simulink model "MultipleAgentsChoice_NoVR"  (R2013b)
settings: Solver=ode45  StartTime=0.0  StopTime=1000  RelTol=1e-4  AbsTol=1e-4
libraries: simulink x24
(part 3 of 5)

== system MultipleAgentsChoice_NoVR/StatePropagation/SatelliteControlAccel/Agent Body3/Actual Thruster response ==
  note: UNRELIABLE THRUSTER?
  Signals : Inport
  AgentNumber : Inport  Port=2
  Bus Creator{,1..3} (4 alike) : BusCreator  Inputs=3
  Bus Creator4 : BusCreator
  Bus Selector : BusSelector  OutputSignals=A3ControlSignals,ConfigurationSignals.XValves1,ConfigurationSignals.XSwitch1,ConfigurationSignals.YValves,ConfigurationSignals.YSwitch,ConfigurationSignals.ZValves,ConfigurationSignals.ZSwitch,ConfigurationSignals.XYZValves,ConfigurationSignals.XYZSwitch,ConfigurationSignals.A3Break
  Bus Selector1 : BusSelector  OutputSignals=signal1.L1Vent,signal1.L2Vent,signal2.L1Vent,signal2.L2Vent,signal3.L1Vent,signal3.L2Vent,XYZ.L1Vent,XYZ.L2Vent  OutputAsBus=on
  Constant{,1..3} (4 alike) : Constant
  Conv2XYZ : MATLABFcn  MATLABFcn=Conv2XYZ_multi  OutputDimensions=3
  Demux : Demux
  Derivative : Derivative
  Mux : Mux  Inputs=5
  Mux1 : Mux  Inputs=2
  PressureTank : Subsystem
  Reliable : Constant
  Sum : Sum  Inputs=|++
  Switch : ManualSwitch
  ThrusterSuiteNumber1 : Constant  Value=4
  Unreliable : Constant  Value=0
  VentForce : MATLABFcn  MATLABFcn=VentForce_multi  OutputDimensions=3
  XYZthruster : Subsystem
  Xthruster : Subsystem
  Ythruster1 : Subsystem
  Zthruster1 : Subsystem
  XThrusterData : Outport
  YThrusterData : Outport  Port=2
  ZThrusterData : Outport  Port=3
  XYZThrusterData : Outport  Port=4
  Forces : Outport  Port=5
  PressureData : Outport  Port=6
  wires:
  Derivative/1 -> Mux1/2  "MainTankDerrivative"
  [NumThrusters] -> PressureTank/1(NumThrusters)
  [FeedPressure] -> XYZthruster/1(FeedPressure)
  [FeedPressure] -> Zthruster1/1(FeedPressure)
  [FeedPressure] -> Ythruster1/1(FeedPressure)
  [FeedPressure] -> Xthruster/1(FeedPressure)
  Ythruster1/3(ActivityData) -> [VentY]
  Zthruster1/3(Activitydata) -> [VentZ]
  XYZthruster/3(Activitydata) -> [VentXYZ]
  Xthruster/3(ActivityData) -> [VentX]
  [VentX] -> Bus Creator4/1
  [VentXYZ] -> Bus Creator4/4
  [VentZ] -> Bus Creator4/3
  [VentY] -> Bus Creator4/2
  ThrusterSuiteNumber1/1 -> [NumThrusters]
  PressureTank/1(TankPressure) -> Mux1/1, Derivative/1, [FeedPressure]  "MainTankPressure"
  Bus Creator4/1 -> PressureTank/2(GroupVentData), Bus Selector1/1
  Mux1/1 -> PressureData/1
  AgentNumber/1 -> Mux/5
  Constant3/1 -> Bus Creator/1
  Signals/1 -> Bus Selector/1
  Mux/1 -> Conv2XYZ/1
  Bus Selector/1 -> Demux/1  "<A3ControlSignals>"
  Demux/1 -> Xthruster/2(ForceRequest)
  Xthruster/2(Xforces) -> Mux/1
  Bus Selector/5 -> Bus Creator1/3  "<YSwitch>"
  Bus Selector/6 -> Bus Creator2/2  "<ZValves>"
  Bus Selector/7 -> Bus Creator2/3  "<ZSwitch>"
  Demux/2 -> Ythruster1/2(ForceRequest)
  Demux/3 -> Zthruster1/2(ForceRequest)
  Ythruster1/2(Yforces) -> Mux/2
  Xthruster/1(XData) -> XThrusterData/1  "A3XThrusterData"
  Ythruster1/1(YData) -> YThrusterData/1  "A3YThrusterData"
  Zthruster1/1(ZData) -> ZThrusterData/1  "A3ZThrusterData"
  Bus Creator/1 -> Xthruster/3(Data)
  Bus Selector/2 -> Bus Creator/2  "<XValves1>"
  Bus Selector/3 -> Bus Creator/3  "<XSwitch1>"
  Constant/1 -> Bus Creator1/1
  Bus Creator1/1 -> Ythruster1/3(Data)
  Constant1/1 -> Bus Creator2/1
  Bus Creator2/1 -> Zthruster1/3(Data)
  Zthruster1/2(Zforces) -> Mux/3
  Bus Selector/4 -> Bus Creator1/2  "<YValves>"
  XYZthruster/1(XYZData) -> XYZThrusterData/1  "A3XYZThrusterData"
  XYZthruster/2(XYZforces) -> Mux/4
  Demux/4 -> XYZthruster/2(ForceRequest)
  Constant2/1 -> Bus Creator3/1
  Bus Creator3/1 -> XYZthruster/3(Data)
  Bus Selector/8 -> Bus Creator3/2  "<XYZValves>"
  Bus Selector/9 -> Bus Creator3/3  "<XYZSwitch>"
  Unreliable/1 -> Switch/2
  Reliable/1 -> Switch/1
  Switch/1 -> Zthruster1/4(Reliability)
  Bus Selector/10 -> Zthruster1/5(BrokenLine)  "<A3Break>"
  VentForce/1 -> Sum/1
  Sum/1 -> Forces/1
  Conv2XYZ/1 -> Sum/2
  Bus Selector1/1 -> VentForce/1

== system MultipleAgentsChoice_NoVR/StatePropagation/SatelliteControlAccel/Agent Body3/Convert2Accels ==
  note: convert forces to accelerations based on 20kg mass and conv to km units
  Forces : Inport
  Conv KM : Gain  Gain=0.001
  mass : Gain  Gain=0.05
  Accels : Outport
  wires:
  Forces/1 -> mass/1
  Conv KM/1 -> Accels/1
  mass/1 -> Conv KM/1

== system MultipleAgentsChoice_NoVR/StatePropagation/SatelliteControlAccel/GetCmdAIL/Triggered run ==
  Trigger : TriggerPort
  DimentionsOut1 : Constant  Value=127
  GetCmdAILXYZ : MATLABFcn  MATLABFcn=GetCmdAIL  OutputDimensions=127
  Commands : Outport
  wires:
  DimentionsOut1/1 -> GetCmdAILXYZ/1
  GetCmdAILXYZ/1 -> Commands/1

== system MultipleAgentsChoice_NoVR/StatePropagation/SatelliteControlAccel/Selective Hill State Provision and Discretisation/Agent1 ==
  GEOC_Current : Inport
  LeadAgent : Inport  Port=2
  Bus Creator : BusCreator  Inputs=5
  Bus Selector2 : BusSelector  OutputSignals=Agent1Pos,Agent1Vel,Agent2Pos,Agent2Vel,Agent3Pos,Agent3Vel
  Demux : Demux  Outputs=7
  Hill State multi : MATLABFcn  MATLABFcn=HillErrors_multi  OutputDimensions=7
  Multiport Switch : MultiPortSwitch
  Mux1 : Mux  Inputs=3
  Mux2 : Mux  Inputs=3
  Mux{3..6} (4 alike) : Mux  Inputs=2
  Zero-Order Hold3 : ZeroOrderHold  SampleTime=0.5
  Zero-Order Hold4 : ZeroOrderHold  SampleTime=0.5
  Agent1 : Outport
  wires:
  Mux1/1 -> Zero-Order Hold4/1, Bus Creator/3  "HillVelCont"
  Mux2/1 -> Zero-Order Hold3/1, Bus Creator/2  "HillPosCont"
  Demux/2 -> Mux2/1
  Demux/4 -> Mux2/3
  Demux/3 -> Mux2/2
  Demux/7 -> Mux1/3
  Demux/5 -> Mux1/1
  Demux/6 -> Mux1/2
  Hill State multi/1 -> Demux/1
  LeadAgent/1 -> Multiport Switch/1
  GEOC_Current/1 -> Bus Selector2/1
  Demux/1 -> Bus Creator/1  "HillMagCont"
  Bus Creator/1 -> Agent1/1  "A1HillState"
  Mux3/1 -> Hill State multi/1
  Bus Selector2/1 -> Mux4/1  "<Agent1Pos>"
  Bus Selector2/2 -> Mux4/2  "<Agent1Vel>"
  Bus Selector2/3 -> Mux5/1  "<Agent2Pos>"
  Bus Selector2/4 -> Mux5/2  "<Agent2Vel>"
  Bus Selector2/5 -> Mux6/1  "<Agent3Pos>"
  Bus Selector2/6 -> Mux6/2  "<Agent3Vel>"
  Mux4/1 -> [Agent1]
  Mux5/1 -> [Agent2]
  Mux6/1 -> [Agent3]
  Multiport Switch/1 -> Mux3/2
  [Agent1] -> Multiport Switch/2
  [Agent2] -> Multiport Switch/3
  [Agent3] -> Multiport Switch/4
  [Agent1] -> Mux3/1
  Zero-Order Hold4/1 -> Bus Creator/5  "HillVelDisc"
  Zero-Order Hold3/1 -> Bus Creator/4  "HillPosDisc"

== system MultipleAgentsChoice_NoVR/StatePropagation/SatelliteControlAccel/Selective Hill State Provision and Discretisation/Agent2 ==
  GEOC_Current : Inport
  LeadAgent : Inport  Port=2
  Bus Creator : BusCreator  Inputs=5
  Bus Selector2 : BusSelector  OutputSignals=Agent1Pos,Agent1Vel,Agent2Pos,Agent2Vel,Agent3Pos,Agent3Vel
  Demux : Demux  Outputs=7
  Hill State multi : MATLABFcn  MATLABFcn=HillErrors_multi  OutputDimensions=7
  Multiport Switch : MultiPortSwitch
  Mux1 : Mux  Inputs=3
  Mux2 : Mux  Inputs=3
  Mux{3..6} (4 alike) : Mux  Inputs=2
  Zero-Order Hold3 : ZeroOrderHold  SampleTime=0.5
  Zero-Order Hold4 : ZeroOrderHold  SampleTime=0.5
  Agent2 : Outport
  wires:
  [Agent3] -> Multiport Switch/4
  [Agent2] -> Multiport Switch/3
  [Agent1] -> Multiport Switch/2
  Multiport Switch/1 -> Mux3/2
  Mux6/1 -> [Agent3]
  Mux5/1 -> [Agent2]
  Mux4/1 -> [Agent1]
  Bus Selector2/6 -> Mux6/2  "<Agent3Vel>"
  Bus Selector2/5 -> Mux6/1  "<Agent3Pos>"
  Bus Selector2/4 -> Mux5/2  "<Agent2Vel>"
  Bus Selector2/3 -> Mux5/1  "<Agent2Pos>"
  Bus Selector2/2 -> Mux4/2  "<Agent1Vel>"
  Bus Selector2/1 -> Mux4/1  "<Agent1Pos>"
  [Agent2] -> Mux3/1
  Mux3/1 -> Hill State multi/1
  Bus Creator/1 -> Agent2/1  "A2HillState"
  Demux/1 -> Bus Creator/1  "HillMagCont"
  GEOC_Current/1 -> Bus Selector2/1
  LeadAgent/1 -> Multiport Switch/1
  Hill State multi/1 -> Demux/1
  Demux/6 -> Mux1/2
  Demux/5 -> Mux1/1
  Demux/7 -> Mux1/3
  Demux/3 -> Mux2/2
  Demux/4 -> Mux2/3
  Demux/2 -> Mux2/1
  Mux2/1 -> Zero-Order Hold3/1, Bus Creator/2  "HillPosCont"
  Mux1/1 -> Zero-Order Hold4/1, Bus Creator/3  "HillVelCont"
  Zero-Order Hold3/1 -> Bus Creator/4  "HillPosDisc"
  Zero-Order Hold4/1 -> Bus Creator/5  "HillVelDisc"

== system MultipleAgentsChoice_NoVR/StatePropagation/SatelliteControlAccel/Selective Hill State Provision and Discretisation/Agent3 ==
  GEOC_Current : Inport
  LeadAgent : Inport  Port=2
  Bus Creator : BusCreator  Inputs=5
  Bus Selector2 : BusSelector  OutputSignals=Agent1Pos,Agent1Vel,Agent2Pos,Agent2Vel,Agent3Pos,Agent3Vel
  Demux : Demux  Outputs=7
  Hill State multi : MATLABFcn  MATLABFcn=HillErrors_multi  OutputDimensions=7
  Multiport Switch : MultiPortSwitch
  Mux1 : Mux  Inputs=3
  Mux2 : Mux  Inputs=3
  Mux{3..6} (4 alike) : Mux  Inputs=2
  Zero-Order Hold3 : ZeroOrderHold  SampleTime=0.5
  Zero-Order Hold4 : ZeroOrderHold  SampleTime=0.5
  Agent3 : Outport
  wires:
  Mux1/1 -> Zero-Order Hold4/1, Bus Creator/3  "HillVelCont"
  Mux2/1 -> Zero-Order Hold3/1, Bus Creator/2  "HillPosCont"
  Demux/2 -> Mux2/1
  Demux/4 -> Mux2/3
  Demux/3 -> Mux2/2
  Demux/7 -> Mux1/3
  Demux/5 -> Mux1/1
  Demux/6 -> Mux1/2
  Hill State multi/1 -> Demux/1
  LeadAgent/1 -> Multiport Switch/1
  GEOC_Current/1 -> Bus Selector2/1
  Zero-Order Hold4/1 -> Bus Creator/5  "HillVelDisc"
  Demux/1 -> Bus Creator/1  "HillMagCont"
  Bus Creator/1 -> Agent3/1  "A3HillState"
  Mux3/1 -> Hill State multi/1
  Bus Selector2/1 -> Mux4/1  "<Agent1Pos>"
  Bus Selector2/2 -> Mux4/2  "<Agent1Vel>"
  Bus Selector2/3 -> Mux5/1  "<Agent2Pos>"
  Bus Selector2/4 -> Mux5/2  "<Agent2Vel>"
  Bus Selector2/5 -> Mux6/1  "<Agent3Pos>"
  Bus Selector2/6 -> Mux6/2  "<Agent3Vel>"
  Mux4/1 -> [Agent1]
  Mux5/1 -> [Agent2]
  Mux6/1 -> [Agent3]
  [Agent1] -> Multiport Switch/2
  [Agent2] -> Multiport Switch/3
  [Agent3] -> Multiport Switch/4
  [Agent3] -> Mux3/1
  Multiport Switch/1 -> Mux3/2
  Zero-Order Hold3/1 -> Bus Creator/4  "HillPosDisc"

== system MultipleAgentsChoice_NoVR/StatePropagation/SatelliteControlAccel/Selective Hill State Provision and Discretisation/MemoryUpdate ==
  GEOC_Current : Inport
  LeadAgent : Inport  Port=2
  Bus Selector2 : BusSelector  OutputSignals=Agent1Pos,Agent1Vel,Agent2Pos,Agent2Vel,Agent3Pos,Agent3Vel
  Multiport Switch : MultiPortSwitch
  Mux4 : Mux  Inputs=2
  Mux5 : Mux  Inputs=2
  Mux6 : Mux  Inputs=2
  Updatememory : MATLABFcn  MATLABFcn=UpdateMemory  OutputDimensions=0
  wires:
  Multiport Switch/1 -> Updatememory/1
  Mux6/1 -> Multiport Switch/4
  Mux5/1 -> Multiport Switch/3
  Mux4/1 -> Multiport Switch/2
  Bus Selector2/6 -> Mux6/2  "<Agent3Vel>"
  Bus Selector2/5 -> Mux6/1  "<Agent3Pos>"
  Bus Selector2/4 -> Mux5/2  "<Agent2Vel>"
  Bus Selector2/3 -> Mux5/1  "<Agent2Pos>"
  Bus Selector2/2 -> Mux4/2  "<Agent1Vel>"
  Bus Selector2/1 -> Mux4/1  "<Agent1Pos>"
  GEOC_Current/1 -> Bus Selector2/1
  LeadAgent/1 -> Multiport Switch/1

== system MultipleAgentsChoice_NoVR/StatePropagation/SatelliteControlAccel/TriggeredSendAgent/SendToAIL ==
  A1ActualForces : Inport
  A1PlanMsg : Inport  Port=2
  A1DesiredForces : Inport  Port=3
  A1StateInfo : Inport  Port=4
  A1tank : Inport  Port=5
  A1XThruster : Inport  Port=6
  A1YThruster : Inport  Port=7
  A1ZThruster : Inport  Port=8
  A1XYZThruster : Inport  Port=9
  A2ActualForces : Inport  Port=10
  A2PlanMsg : Inport  Port=11
  A2DesiredForces : Inport  Port=12
  A2StateInfo : Inport  Port=13
  A2tank : Inport  Port=14
  A2XThruster : Inport  Port=15
  A2YThruster : Inport  Port=16
  A2ZThruster : Inport  Port=17
  A2XYZThruster : Inport  Port=18
  A3ActualForces : Inport  Port=19
  A3PlanMsg : Inport  Port=20
  A3DesiredForces : Inport  Port=21
  A3StateInfo : Inport  Port=22
  A3tank : Inport  Port=23
  A3XThruster : Inport  Port=24
  A3YThruster : Inport  Port=25
  A3ZThruster : Inport  Port=26
  A3XYZThruster : Inport  Port=27
  Display : Display
  MATLAB Fcn : MATLABFcn  MATLABFcn=CommunicateWithTagsMulti  OutputDimensions=0
  Mux : Mux  Inputs=27
  wires:
  A1ActualForces/1 -> Mux/1  "A1ActualForces"
  A1PlanMsg/1 -> Mux/2  "A1PlanMsg"
  A1StateInfo/1 -> Mux/4  "A1StateInfo"
  A1XThruster/1 -> Mux/6  "A1XThruster"
  A1YThruster/1 -> Mux/7  "A1YThruster"
  A1ZThruster/1 -> Mux/8  "A1ZThruster"
  A1DesiredForces/1 -> Mux/3  "A1DesiredForfces"
  A1tank/1 -> Mux/5  "A1Tank"
  A2ActualForces/1 -> Mux/10  "A2ActualForces"
  A2PlanMsg/1 -> Mux/11  "A2PlanMsg"
  A2StateInfo/1 -> Mux/13  "A2StateInfo"
  A2XThruster/1 -> Mux/15  "A2XThruster"
  A2YThruster/1 -> Mux/16  "A2YThruster"
  A2ZThruster/1 -> Mux/17  "A2ZThruster"
  A2DesiredForces/1 -> Mux/12  "A2DesiredForces"
  A2tank/1 -> Mux/14  "A2Tank"
  A1XYZThruster/1 -> Mux/9  "A1XYZThruster"
  A2XYZThruster/1 -> Mux/18  "A2XYZThruster"
  A3PlanMsg/1 -> Mux/20  "A3PlanMsg"
  A3DesiredForces/1 -> Mux/21  "A3DesiredForces"
  A3StateInfo/1 -> Mux/22  "A3StateInfo"
  A3tank/1 -> Mux/23  "A3Tank"
  A3XThruster/1 -> Mux/24  "A3XThruster"
  A3YThruster/1 -> Mux/25  "A3YThruster"
  A3ZThruster/1 -> Mux/26  "A3ZThruster"
  A3XYZThruster/1 -> Mux/27  "A3XYZThruster"
  A3ActualForces/1 -> Mux/19  "A3ActualForces"
  Mux/1 -> MATLAB Fcn/1, Display/1

== system MultipleAgentsChoice_NoVR/StatePropagation/SatelliteControlAccel/TriggeredSendCont/SendToCont ==
  A1ActualForces : Inport
  A1PlanMsg : Inport  Port=2
  A1DesiredForces : Inport  Port=3
  A1StateInfo : Inport  Port=4
  A1tank : Inport  Port=5
  A1XThruster : Inport  Port=6
  A1YThruster : Inport  Port=7
  A1ZThruster : Inport  Port=8
  A1XYZThruster : Inport  Port=9
  A2ActualForces : Inport  Port=10
  A2PlanMsg : Inport  Port=11
  A2DesiredForces : Inport  Port=12
  A2StateInfo : Inport  Port=13
  A2tank : Inport  Port=14
  A2XThruster : Inport  Port=15
  A2YThruster : Inport  Port=16
  A2ZThruster : Inport  Port=17
  A2XYZThruster : Inport  Port=18
  A3ActualForces : Inport  Port=19
  A3PlanMsg : Inport  Port=20
  A3DesiredForces : Inport  Port=21
  A3StateInfo : Inport  Port=22
  A3tank : Inport  Port=23
  A3XThruster : Inport  Port=24
  A3YThruster : Inport  Port=25
  A3ZThruster : Inport  Port=26
  A3XYZThruster : Inport  Port=27
  Display : Display
  MATLAB Fcn : MATLABFcn  MATLABFcn=CommunicateWithCont  OutputDimensions=0
  Mux : Mux  Inputs=27
  wires:
  Mux/1 -> Display/1, MATLAB Fcn/1
  A3ActualForces/1 -> Mux/19  "A3ActualForces"
  A3XYZThruster/1 -> Mux/27  "A3XYZThruster"
  A3ZThruster/1 -> Mux/26  "A3ZThruster"
  A3YThruster/1 -> Mux/25  "A3YThruster"
  A3XThruster/1 -> Mux/24  "A3XThruster"
  A3tank/1 -> Mux/23  "A3tank"
  A3StateInfo/1 -> Mux/22  "A3StateInfo"
  A3DesiredForces/1 -> Mux/21  "A3DesiredForces"
  A3PlanMsg/1 -> Mux/20  "A3PlanMsg"
  A2XYZThruster/1 -> Mux/18  "A2XYZThruster"
  A1XYZThruster/1 -> Mux/9  "A1XYZThruster"
  A2tank/1 -> Mux/14  "A2tank"
  A2DesiredForces/1 -> Mux/12  "A2DesiredForces"
  A2ZThruster/1 -> Mux/17  "A2ZThruster"
  A2YThruster/1 -> Mux/16  "A2YThruster"
  A2XThruster/1 -> Mux/15  "A2XThruster"
  A2StateInfo/1 -> Mux/13  "A2StateInfo"
  A2PlanMsg/1 -> Mux/11  "A2PlanMsg"
  A2ActualForces/1 -> Mux/10  "A2ActualForces"
  A1tank/1 -> Mux/5  "A1tank"
  A1DesiredForces/1 -> Mux/3  "A1DesiredForfces"
  A1ZThruster/1 -> Mux/8  "A1ZThruster"
  A1YThruster/1 -> Mux/7  "A1YThruster"
  A1XThruster/1 -> Mux/6  "A1XThruster"
  A1StateInfo/1 -> Mux/4  "A1StateInfo"
  A1PlanMsg/1 -> Mux/2  "A1PlanMsg"
  A1ActualForces/1 -> Mux/1  "A1ActualForces"

== system MultipleAgentsChoice_NoVR/StatePropagation/SatelliteControlAccel/Agent Body1/Actual Thruster response/PressureTank ==
  NumThrusters : Inport
  GroupVentData : Inport  Port=2
  Clock : Clock
  Display : Display
  DropRate : MATLABFcn  MATLABFcn=DropRate_multi  OutputDimensions=1
  Integrator : Integrator  InitialConditionSource=external
  Mux : Mux  Inputs=2
  Start : Constant  Value=0
  StartPressure : Constant  Value=100
  Switch1 : Switch
  TankPressure : Outport
  wires:
  DropRate/1 -> Switch1/1
  Mux/1 -> DropRate/1
  NumThrusters/1 -> Mux/1
  GroupVentData/1 -> Mux/2
  Switch1/1 -> Integrator/1
  Clock/1 -> Switch1/2
  Start/1 -> Switch1/3
  Integrator/1 -> Display/1, TankPressure/1
  StartPressure/1 -> Integrator/2

== system MultipleAgentsChoice_NoVR/StatePropagation/SatelliteControlAccel/Agent Body1/Actual Thruster response/XYZthruster ==
  note: NB:-Agent has no knowledge of red blocks
      |             -Blue blocks prescribed by agent
  note: Tank pressure and thruster selection: must declare number of thrusters
  FeedPressure : Inport
  ForceRequest : Inport  Port=2
  Data : Inport  Port=3
  Bus Creator2 : BusCreator  Inputs=3
  Bus Selector : BusSelector  OutputSignals=XYZValves,XYZSwitch
  Constant : Constant
  Constant1 : Constant  Value=0
  Switch : Switch  Criteria=u2 ~= 0
  Thruster1 : Subsystem
  XYZData : Outport
  XYZforces : Outport  Port=2
  Activitydata : Outport  Port=3
  wires:
  ForceRequest/1 -> Thruster1/4(ForceRequest)  "XYZforces"
  Thruster1/1(L1Vent) -> Bus Creator2/1  "L1Vent"
  Thruster1/2(L2Vent) -> Bus Creator2/2  "L2Vent"
  FeedPressure/1 -> Thruster1/2(FeedPressure)
  Constant/1 -> Switch/1
  Constant1/1 -> Switch/3
  Thruster1/4(thrusterData) -> XYZData/1  "A1TXYZ1"
  Data/1 -> Bus Selector/1
  Bus Selector/1 -> Thruster1/1(ValveAssign)  "<XYZValves>"
  Bus Selector/2 -> Thruster1/3(MainSwitch)  "<XYZSwitch>"
  Thruster1/3(Forces) -> XYZforces/1, Switch/2
  Switch/1 -> Bus Creator2/3  "Active1"
  Bus Creator2/1 -> Activitydata/1  "XYZ"

== system MultipleAgentsChoice_NoVR/StatePropagation/SatelliteControlAccel/Agent Body1/Actual Thruster response/Xthruster ==
  note: Tank pressure and thruster selection: must declare number of thrusters
  note: NB:-Agent has no knowledge of red blocks
      |             -Blue blocks prescribed by agent
  FeedPressure : Inport
  ForceRequest : Inport  Port=2
  Data : Inport  Port=3
  Bus Creator2 : BusCreator  Inputs=3
  Bus Selector : BusSelector  OutputSignals=XValves1,XSwitch1
  Constant : Constant
  Constant1 : Constant  Value=0
  Switch : Switch  Criteria=u2 ~= 0
  Thruster1 : Subsystem
  XData : Outport
  Xforces : Outport  Port=2
  ActivityData : Outport  Port=3
  wires:
  Bus Creator2/1 -> ActivityData/1
  Switch/1 -> Bus Creator2/3  "Active1"
  Thruster1/3(Forces) -> Xforces/1, Switch/2
  Bus Selector/2 -> Thruster1/3(MainSwitch)  "<XSwitch1>"
  Bus Selector/1 -> Thruster1/1(ValveAssign)  "<XValves1>"
  Data/1 -> Bus Selector/1
  Thruster1/4(ThrusterData) -> XData/1
  Constant1/1 -> Switch/3
  Constant/1 -> Switch/1
  FeedPressure/1 -> Thruster1/2(FeedPressure)
  Thruster1/2(L2Vent) -> Bus Creator2/2  "L2Vent"
  Thruster1/1(L1Vent) -> Bus Creator2/1  "L1Vent"
  ForceRequest/1 -> Thruster1/4(ForceRequest)  "Xforces"

== system MultipleAgentsChoice_NoVR/StatePropagation/SatelliteControlAccel/Agent Body1/Actual Thruster response/Ythruster1 ==
  note: NB:-Agent has no knowledge of red blocks
      |             -Blue blocks prescribed by agent
  note: Tank pressure and thruster selection: must declare number of thrusters
  FeedPressure : Inport
  ForceRequest : Inport  Port=2
  Data : Inport  Port=3
  Bus Creator2 : BusCreator  Inputs=3
  Bus Selector : BusSelector  OutputSignals=YValves,YSwitch
  Constant : Constant
  Constant1 : Constant  Value=0
  Switch : Switch  Criteria=u2 ~= 0
  Thruster1 : Subsystem
  YData : Outport
  Yforces : Outport  Port=2
  ActivityData : Outport  Port=3
  wires:
  ForceRequest/1 -> Thruster1/4(ForceRequest)  "Yforces"
  Thruster1/1(L1Vent) -> Bus Creator2/1  "L1Vent"
  Thruster1/2(L2Vent) -> Bus Creator2/2  "L2Vent"
  [ValveAssign1] -> Thruster1/1(ValveAssign)
  [MainSwitch1] -> Thruster1/3(MainSwitch)
  FeedPressure/1 -> Thruster1/2(FeedPressure)
  Constant/1 -> Switch/1
  Constant1/1 -> Switch/3
  Thruster1/4(thrusterData) -> YData/1  "A1TY1"
  Data/1 -> Bus Selector/1
  Bus Selector/1 -> [ValveAssign1]  "<YValves>"
  Bus Selector/2 -> [MainSwitch1]  "<YSwitch>"
  Thruster1/3(Forces) -> Yforces/1, Switch/2
  Switch/1 -> Bus Creator2/3  "Active1"
  Bus Creator2/1 -> ActivityData/1

== system MultipleAgentsChoice_NoVR/StatePropagation/SatelliteControlAccel/Agent Body1/Actual Thruster response/Zthruster1 ==
  note: Tank pressure and thruster selection: must declare number of thrusters
  note: NB:-Agent has no knowledge of red blocks
      |             -Blue blocks prescribed by agent
  FeedPressure : Inport
  ForceRequest : Inport  Port=2
  Data : Inport  Port=3
  Reliability : Inport  Port=4
  BrokenLine : Inport  Port=5
  Bus Creator2 : BusCreator  Inputs=3
  Bus Selector : BusSelector  OutputSignals=ZValves,ZSwitch
  Constant : Constant
  Constant1 : Constant  Value=0
  Switch : Switch  Criteria=u2 ~= 0
  Thruster1 : Subsystem
  ZData : Outport
  Zforces : Outport  Port=2
  Activitydata : Outport  Port=3
  wires:
  Reliability/1 -> Thruster1/5(Reliability)
  Bus Creator2/1 -> Activitydata/1
  Switch/1 -> Bus Creator2/3  "Active1"
  Thruster1/3(Forces) -> Switch/2, Zforces/1
  Bus Selector/2 -> Thruster1/3(MainSwitch)  "<ZSwitch>"
  Bus Selector/1 -> Thruster1/1(ValveAssign)  "<ZValves>"
  Data/1 -> Bus Selector/1
  Thruster1/4(thrusterData) -> ZData/1  "A1TZ1"
  Constant1/1 -> Switch/3
  Constant/1 -> Switch/1
  FeedPressure/1 -> Thruster1/2(FeedPressure)
  Thruster1/2(L2Vent) -> Bus Creator2/2  "L2Vent"
  Thruster1/1(L1Vent) -> Bus Creator2/1  "L1Vent"
  ForceRequest/1 -> Thruster1/4(ForceRequest)  "Zforces"
  BrokenLine/1 -> Thruster1/6(BrokenLine)

== system MultipleAgentsChoice_NoVR/StatePropagation/SatelliteControlAccel/Agent Body2/Actual Thruster response/PressureTank ==
  NumThrusters : Inport
  GroupVentData : Inport  Port=2
  Clock : Clock
  Display : Display
  DropRate : MATLABFcn  MATLABFcn=DropRate_multi  OutputDimensions=1
  Integrator : Integrator  InitialConditionSource=external
  Mux : Mux  Inputs=2
  Start : Constant  Value=0
  StartPressure : Constant  Value=100
  Switch1 : Switch
  TankPressure : Outport
  wires:
  StartPressure/1 -> Integrator/2
  Integrator/1 -> TankPressure/1, Display/1
  Start/1 -> Switch1/3
  Clock/1 -> Switch1/2
  Switch1/1 -> Integrator/1
  GroupVentData/1 -> Mux/2
  NumThrusters/1 -> Mux/1
  Mux/1 -> DropRate/1
  DropRate/1 -> Switch1/1

== system MultipleAgentsChoice_NoVR/StatePropagation/SatelliteControlAccel/Agent Body2/Actual Thruster response/XYZthruster ==
  note: Tank pressure and thruster selection: must declare number of thrusters
  note: NB:-Agent has no knowledge of red blocks
      |             -Blue blocks prescribed by agent
  FeedPressure : Inport
  ForceRequest : Inport  Port=2
  Data : Inport  Port=3
  Bus Creator2 : BusCreator  Inputs=3
  Bus Selector : BusSelector  OutputSignals=XYZValves,XYZSwitch
  Constant : Constant
  Constant1 : Constant  Value=0
  Switch : Switch  Criteria=u2 ~= 0
  Thruster1 : Subsystem
  XYZData : Outport
  XYZforces : Outport  Port=2
  Activitydata : Outport  Port=3
  wires:
  Bus Creator2/1 -> Activitydata/1  "XYZ"
  Switch/1 -> Bus Creator2/3  "Active1"
  Thruster1/3(Forces) -> Switch/2, XYZforces/1
  Bus Selector/2 -> Thruster1/3(MainSwitch)  "<XYZSwitch>"
  Bus Selector/1 -> Thruster1/1(ValveAssign)  "<XYZValves>"
  Data/1 -> Bus Selector/1
  Thruster1/4(thrusterData) -> XYZData/1
  Constant1/1 -> Switch/3
  Constant/1 -> Switch/1
  FeedPressure/1 -> Thruster1/2(FeedPressure)
  Thruster1/2(L2Vent) -> Bus Creator2/2  "L2Vent"
  Thruster1/1(L1Vent) -> Bus Creator2/1  "L1Vent"
  ForceRequest/1 -> Thruster1/4(ForceRequest)  "XYZforces"

== system MultipleAgentsChoice_NoVR/StatePropagation/SatelliteControlAccel/Agent Body2/Actual Thruster response/Xthruster ==
  note: NB:-Agent has no knowledge of red blocks
      |             -Blue blocks prescribed by agent
  note: Tank pressure and thruster selection: must declare number of thrusters
  FeedPressure : Inport
  ForceRequest : Inport  Port=2
  Data : Inport  Port=3
  Bus Creator2 : BusCreator  Inputs=3
  Bus Selector : BusSelector  OutputSignals=XValves1,XSwitch1
  Constant : Constant
  Constant1 : Constant  Value=0
  Switch : Switch  Criteria=u2 ~= 0
  Thruster1 : Subsystem
  XData : Outport
  Xforces : Outport  Port=2
  ActivityData : Outport  Port=3
  wires:
  ForceRequest/1 -> Thruster1/4(ForceRequest)  "Xforces"
  Thruster1/1(L1Vent) -> Bus Creator2/1  "L1Vent"
  Thruster1/2(L2Vent) -> Bus Creator2/2  "L2Vent"
  FeedPressure/1 -> Thruster1/2(FeedPressure)
  Constant/1 -> Switch/1
  Constant1/1 -> Switch/3
  Thruster1/4(ThrusterData) -> XData/1  "A2TX"
  Data/1 -> Bus Selector/1
  Bus Selector/1 -> Thruster1/1(ValveAssign)  "<XValves1>"
  Bus Selector/2 -> Thruster1/3(MainSwitch)  "<XSwitch1>"
  Thruster1/3(Forces) -> Switch/2, Xforces/1
  Switch/1 -> Bus Creator2/3  "Active1"
  Bus Creator2/1 -> ActivityData/1

== system MultipleAgentsChoice_NoVR/StatePropagation/SatelliteControlAccel/Agent Body2/Actual Thruster response/Ythruster1 ==
  note: Tank pressure and thruster selection: must declare number of thrusters
  note: NB:-Agent has no knowledge of red blocks
      |             -Blue blocks prescribed by agent
  FeedPressure : Inport
  ForceRequest : Inport  Port=2
  Data : Inport  Port=3
  Bus Creator2 : BusCreator  Inputs=3
  Bus Selector : BusSelector  OutputSignals=YValves,YSwitch
  Constant : Constant
  Constant1 : Constant  Value=0
  Switch : Switch  Criteria=u2 ~= 0
  Thruster1 : Subsystem
  YData : Outport
  Yforces : Outport  Port=2
  ActivityData : Outport  Port=3
  wires:
  Bus Creator2/1 -> ActivityData/1
  Switch/1 -> Bus Creator2/3  "Active1"
  Thruster1/3(Forces) -> Switch/2, Yforces/1
  Bus Selector/2 -> [MainSwitch1]  "<YSwitch>"
  Bus Selector/1 -> [ValveAssign1]  "<YValves>"
  Data/1 -> Bus Selector/1
  Thruster1/4(thrusterData) -> YData/1  "A2TY"
  Constant1/1 -> Switch/3
  Constant/1 -> Switch/1
  FeedPressure/1 -> Thruster1/2(FeedPressure)
  [MainSwitch1] -> Thruster1/3(MainSwitch)
  [ValveAssign1] -> Thruster1/1(ValveAssign)
  Thruster1/2(L2Vent) -> Bus Creator2/2  "L2Vent"
  Thruster1/1(L1Vent) -> Bus Creator2/1  "L1Vent"
  ForceRequest/1 -> Thruster1/4(ForceRequest)  "Yforces"

== system MultipleAgentsChoice_NoVR/StatePropagation/SatelliteControlAccel/Agent Body2/Actual Thruster response/Zthruster1 ==
  note: NB:-Agent has no knowledge of red blocks
      |             -Blue blocks prescribed by agent
  note: Tank pressure and thruster selection: must declare number of thrusters
  FeedPressure : Inport
  ForceRequest : Inport  Port=2
  Data : Inport  Port=3
  Reliability : Inport  Port=4
  BrokenLine : Inport  Port=5
  Bus Creator2 : BusCreator  Inputs=3
  Bus Selector : BusSelector  OutputSignals=ZValves,ZSwitch
  Constant : Constant
  Constant1 : Constant  Value=0
  Switch : Switch  Criteria=u2 ~= 0
  Thruster1 : Subsystem
  ZData : Outport
  Zforces : Outport  Port=2
  Activitydata : Outport  Port=3
  wires:
  ForceRequest/1 -> Thruster1/4(ForceRequest)  "Zforces"
  Thruster1/1(L1Vent) -> Bus Creator2/1  "L1Vent"
  Thruster1/2(L2Vent) -> Bus Creator2/2  "L2Vent"
  FeedPressure/1 -> Thruster1/2(FeedPressure)
  Constant/1 -> Switch/1
  Constant1/1 -> Switch/3
  Thruster1/4(thrusterData) -> ZData/1  "A2TZ"
  Data/1 -> Bus Selector/1
  Bus Selector/1 -> Thruster1/1(ValveAssign)  "<ZValves>"
  Bus Selector/2 -> Thruster1/3(MainSwitch)  "<ZSwitch>"
  Thruster1/3(Forces) -> Zforces/1, Switch/2
  Switch/1 -> Bus Creator2/3  "Active1"
  Bus Creator2/1 -> Activitydata/1
  Reliability/1 -> Thruster1/5(Reliability)
  BrokenLine/1 -> Thruster1/6(BrokenLine)

== system MultipleAgentsChoice_NoVR/StatePropagation/SatelliteControlAccel/Agent Body3/Actual Thruster response/PressureTank ==
  NumThrusters : Inport
  GroupVentData : Inport  Port=2
  Clock : Clock
  Display : Display
  DropRate : MATLABFcn  MATLABFcn=DropRate_multi  OutputDimensions=1
  Integrator : Integrator  InitialConditionSource=external
  Mux : Mux  Inputs=2
  Start : Constant  Value=0
  StartPressure : Constant  Value=100
  Switch1 : Switch
  TankPressure : Outport
  wires:
  StartPressure/1 -> Integrator/2
  Integrator/1 -> TankPressure/1, Display/1
  Start/1 -> Switch1/3
  Clock/1 -> Switch1/2
  Switch1/1 -> Integrator/1
  GroupVentData/1 -> Mux/2
  NumThrusters/1 -> Mux/1
  Mux/1 -> DropRate/1
  DropRate/1 -> Switch1/1

== system MultipleAgentsChoice_NoVR/StatePropagation/SatelliteControlAccel/Agent Body3/Actual Thruster response/XYZthruster ==
  note: Tank pressure and thruster selection: must declare number of thrusters
  note: NB:-Agent has no knowledge of red blocks
      |             -Blue blocks prescribed by agent
  FeedPressure : Inport
  ForceRequest : Inport  Port=2
  Data : Inport  Port=3
  Bus Creator2 : BusCreator  Inputs=3
  Bus Selector : BusSelector  OutputSignals=XYZValves,XYZSwitch
  Constant : Constant
  Constant1 : Constant  Value=0
  Switch : Switch  Criteria=u2 ~= 0
  Thruster1 : Subsystem
  XYZData : Outport
  XYZforces : Outport  Port=2
  Activitydata : Outport  Port=3
  wires:
  Bus Creator2/1 -> Activitydata/1  "XYZ"
  Switch/1 -> Bus Creator2/3  "Active1"
  Thruster1/3(Forces) -> Switch/2, XYZforces/1
  Bus Selector/2 -> Thruster1/3(MainSwitch)  "<XYZSwitch>"
  Bus Selector/1 -> Thruster1/1(ValveAssign)  "<XYZValves>"
  Data/1 -> Bus Selector/1
  Thruster1/4(thrusterData) -> XYZData/1  "A3TXYZ"
  Constant1/1 -> Switch/3
  Constant/1 -> Switch/1
  FeedPressure/1 -> Thruster1/2(FeedPressure)
  Thruster1/2(L2Vent) -> Bus Creator2/2  "L2Vent"
  Thruster1/1(L1Vent) -> Bus Creator2/1  "L1Vent"
  ForceRequest/1 -> Thruster1/4(ForceRequest)  "XYZforces"

== system MultipleAgentsChoice_NoVR/StatePropagation/SatelliteControlAccel/Agent Body3/Actual Thruster response/Xthruster ==
  note: NB:-Agent has no knowledge of red blocks
      |             -Blue blocks prescribed by agent
  note: Tank pressure and thruster selection: must declare number of thrusters
  FeedPressure : Inport
  ForceRequest : Inport  Port=2
  Data : Inport  Port=3
  Bus Creator2 : BusCreator  Inputs=3
  Bus Selector : BusSelector  OutputSignals=XValves1,XSwitch1
  Constant : Constant
  Constant1 : Constant  Value=0
  Switch : Switch  Criteria=u2 ~= 0
  Thruster1 : Subsystem
  XData : Outport
  Xforces : Outport  Port=2
  ActivityData : Outport  Port=3
  wires:
  ForceRequest/1 -> Thruster1/4(ForceRequest)  "Xforces"
  Thruster1/1(L1Vent) -> Bus Creator2/1  "L1Vent"
  Thruster1/2(L2Vent) -> Bus Creator2/2  "L2Vent"
  FeedPressure/1 -> Thruster1/2(FeedPressure)
  Constant/1 -> Switch/1
  Constant1/1 -> Switch/3
  Thruster1/4(ThrusterData) -> XData/1  "A3TX"
  Data/1 -> Bus Selector/1
  Bus Selector/1 -> Thruster1/1(ValveAssign)  "<XValves1>"
  Bus Selector/2 -> Thruster1/3(MainSwitch)  "<XSwitch1>"
  Thruster1/3(Forces) -> Switch/2, Xforces/1
  Switch/1 -> Bus Creator2/3  "Active1"
  Bus Creator2/1 -> ActivityData/1

== system MultipleAgentsChoice_NoVR/StatePropagation/SatelliteControlAccel/Agent Body3/Actual Thruster response/Ythruster1 ==
  note: Tank pressure and thruster selection: must declare number of thrusters
  note: NB:-Agent has no knowledge of red blocks
      |             -Blue blocks prescribed by agent
  FeedPressure : Inport
  ForceRequest : Inport  Port=2
  Data : Inport  Port=3
  Bus Creator2 : BusCreator  Inputs=3
  Bus Selector : BusSelector  OutputSignals=YValves,YSwitch
  Constant : Constant
  Constant1 : Constant  Value=0
  Switch : Switch  Criteria=u2 ~= 0
  Thruster1 : Subsystem
  YData : Outport
  Yforces : Outport  Port=2
  ActivityData : Outport  Port=3
  wires:
  Bus Creator2/1 -> ActivityData/1
  Switch/1 -> Bus Creator2/3  "Active1"
  Thruster1/3(Forces) -> Switch/2, Yforces/1
  Bus Selector/2 -> [MainSwitch1]  "<YSwitch>"
  Bus Selector/1 -> [ValveAssign1]  "<YValves>"
  Data/1 -> Bus Selector/1
  Thruster1/4(thrusterData) -> YData/1  "A3TY"
  Constant1/1 -> Switch/3
  Constant/1 -> Switch/1
  FeedPressure/1 -> Thruster1/2(FeedPressure)
  [MainSwitch1] -> Thruster1/3(MainSwitch)
  [ValveAssign1] -> Thruster1/1(ValveAssign)
  Thruster1/2(L2Vent) -> Bus Creator2/2  "L2Vent"
  Thruster1/1(L1Vent) -> Bus Creator2/1  "L1Vent"
  ForceRequest/1 -> Thruster1/4(ForceRequest)  "Yforces"

== system MultipleAgentsChoice_NoVR/StatePropagation/SatelliteControlAccel/Agent Body3/Actual Thruster response/Zthruster1 ==
  note: NB:-Agent has no knowledge of red blocks
      |             -Blue blocks prescribed by agent
  note: Tank pressure and thruster selection: must declare number of thrusters
  FeedPressure : Inport
  ForceRequest : Inport  Port=2
  Data : Inport  Port=3
  Reliability : Inport  Port=4
  BrokenLine : Inport  Port=5
  Bus Creator2 : BusCreator  Inputs=3
  Bus Selector : BusSelector  OutputSignals=ZValves,ZSwitch
  Constant : Constant
  Constant1 : Constant  Value=0
  Switch : Switch  Criteria=u2 ~= 0
  Thruster1 : Subsystem
  ZData : Outport
  Zforces : Outport  Port=2
  Activitydata : Outport  Port=3
  wires:
  ForceRequest/1 -> Thruster1/4(ForceRequest)  "Zforces"
  Thruster1/1(L1Vent) -> Bus Creator2/1  "L1Vent"
  Thruster1/2(L2Vent) -> Bus Creator2/2  "L2Vent"
  FeedPressure/1 -> Thruster1/2(FeedPressure)
  Constant/1 -> Switch/1
  Constant1/1 -> Switch/3
  Thruster1/4(thrusterData) -> ZData/1  "A3TZ"
  Data/1 -> Bus Selector/1
  Bus Selector/1 -> Thruster1/1(ValveAssign)  "<ZValves>"
  Bus Selector/2 -> Thruster1/3(MainSwitch)  "<ZSwitch>"
  Thruster1/3(Forces) -> Zforces/1, Switch/2
  Switch/1 -> Bus Creator2/3  "Active1"
  Bus Creator2/1 -> Activitydata/1
  Reliability/1 -> Thruster1/5(Reliability)
  BrokenLine/1 -> Thruster1/6(BrokenLine)

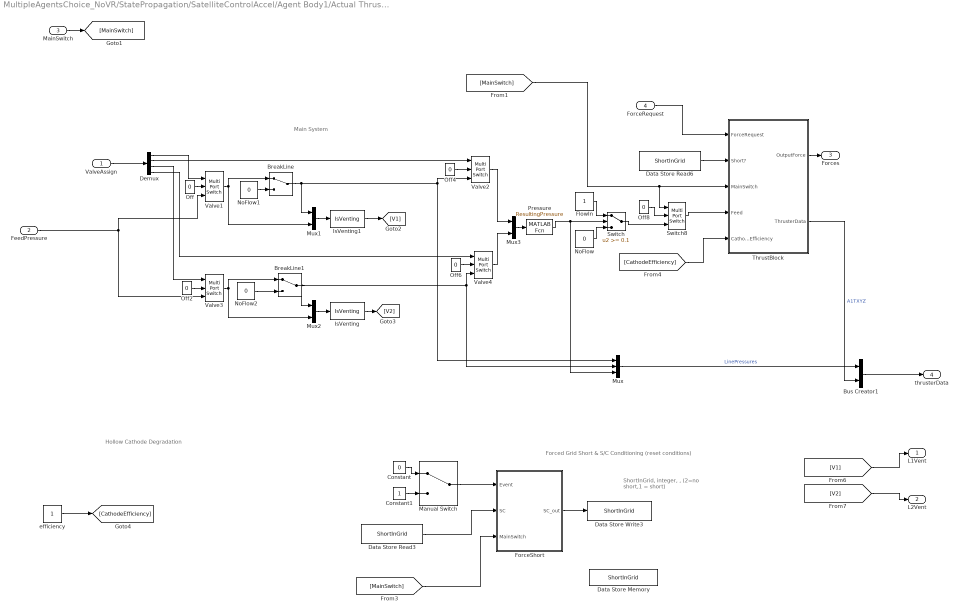
== system MultipleAgentsChoice_NoVR/StatePropagation/SatelliteControlAccel/Agent Body1/Actual Thruster response/XYZthruster/Thruster1 ==
  note: Forced Grid Short & S/C Conditioning (reset conditions)
  note: ShortInGrid, integer, , (2=no short,1 = short)
  note: Hollow Cathode Degradation
  note: Main System
  ValveAssign : Inport
  FeedPressure : Inport  Port=2
  MainSwitch : Inport  Port=3
  ForceRequest : Inport  Port=4
  BreakLine : ManualSwitch
  BreakLine1 : ManualSwitch
  Bus Creator1 : BusCreator  Inputs=2
  Constant : Constant  Value=0
  Constant1 : Constant
  Data Store Memory : DataStoreMemory  DataStoreName=ShortInGrid  ReadBeforeWriteMsg=warning  WriteAfterWriteMsg=warning  WriteAfterReadMsg=warning  InitialValue=2
  Data Store Read3 : DataStoreRead  DataStoreName=ShortInGrid  SampleTime=0
  Data Store Read6 : DataStoreRead  DataStoreName=ShortInGrid  SampleTime=0
  Data Store Write3 : DataStoreWrite  DataStoreName=ShortInGrid
  Demux : Demux
  FlowIn : Constant
  ForceShort : Subsystem
  IsVenting : MATLABFcn  MATLABFcn=IsVenting  OutputDimensions=1
  IsVenting1 : MATLABFcn  MATLABFcn=IsVenting  OutputDimensions=1
  Manual Switch : ManualSwitch
  Mux : Mux  Inputs=3
  Mux1 : Mux  Inputs=2
  Mux2 : Mux  Inputs=2
  Mux3 : Mux  Inputs=2
  NoFlow : Constant  Value=0
  NoFlow1 : Constant  Value=0
  NoFlow2 : Constant  Value=0
  Off{,2,4,6,8} (5 alike) : Constant  Value=0
  Pressure : MATLABFcn  MATLABFcn=ResultingPressure
  Switch : Switch  Threshold=0.1
  Switch8 : MultiPortSwitch  Inputs=2
  ThrustBlock : Subsystem
  Valve{1..4} (4 alike) : MultiPortSwitch  Inputs=2
  efficiency : Constant
  L1Vent : Outport
  L2Vent : Outport  Port=2
  Forces : Outport  Port=3
  thrusterData : Outport  Port=4
  wires:
  ForceShort/1(SC_out) -> Data Store Write3/1
  Constant/1 -> Manual Switch/1
  Constant1/1 -> Manual Switch/2
  Manual Switch/1 -> ForceShort/1(Event)
  Data Store Read3/1 -> ForceShort/2(SC)
  [MainSwitch] -> ForceShort/3(MainSwitch)
  efficiency/1 -> [CathodeEfficiency]
  Valve1/1 -> BreakLine/1, Mux1/2
  Valve2/1 -> Mux3/1
  Mux3/1 -> Pressure/1
  BreakLine/1 -> Mux1/1, Valve2/3, Mux/1
  FlowIn/1 -> Switch/1
  NoFlow/1 -> Switch/3
  Switch8/1 -> ThrustBlock/4(Feed)
  Data Store Read6/1 -> ThrustBlock/2(Short?)
  ValveAssign/1 -> Demux/1
  Demux/1 -> Valve1/1
  Demux/2 -> Valve2/1
  Demux/3 -> Valve3/1
  Demux/4 -> Valve4/1
  ThrustBlock/2(ThrusterData) -> Bus Creator1/2  "A1TXYZ"
  ThrustBlock/1(OutputForce) -> Forces/1
  NoFlow1/1 -> BreakLine/2
  Off/1 -> Valve1/2
  Off4/1 -> Valve2/2
  Off2/1 -> Valve3/2
  Off6/1 -> Valve4/2
  Off8/1 -> Switch8/2
  Switch/1 -> Switch8/3
  Mux/1 -> Bus Creator1/1  "LinePressures"
  NoFlow2/1 -> BreakLine1/2
  Valve3/1 -> BreakLine1/1, Mux2/2
  BreakLine1/1 -> Mux2/1, Valve4/3, Mux/2
  [CathodeEfficiency] -> ThrustBlock/5(CathodeEfficiency)
  ForceRequest/1 -> ThrustBlock/1(ForceRequest)
  Bus Creator1/1 -> thrusterData/1
  Mux1/1 -> IsVenting1/1
  Mux2/1 -> IsVenting/1
  Pressure/1 -> Switch/2, Mux/3
  IsVenting1/1 -> [V1]
  IsVenting/1 -> [V2]
  FeedPressure/1 -> Valve1/3, Valve3/3
  MainSwitch/1 -> [MainSwitch]
  Valve4/1 -> Mux3/2
  [MainSwitch] -> ThrustBlock/3(MainSwitch), Switch8/1
  [V1] -> L1Vent/1
  [V2] -> L2Vent/1

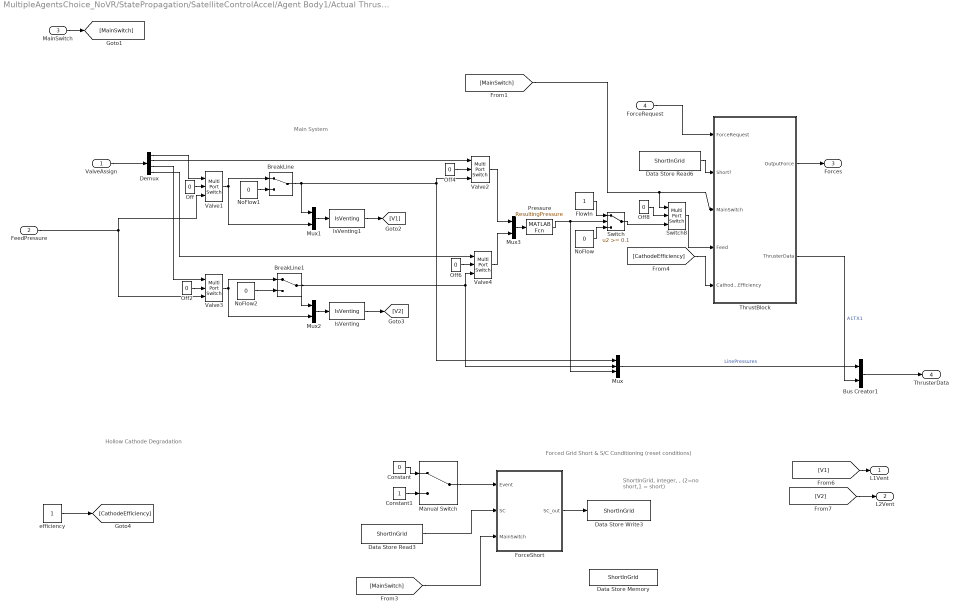
== system MultipleAgentsChoice_NoVR/StatePropagation/SatelliteControlAccel/Agent Body1/Actual Thruster response/Xthruster/Thruster1 ==
  note: Main System
  note: Hollow Cathode Degradation
  note: ShortInGrid, integer, , (2=no short,1 = short)
  note: Forced Grid Short & S/C Conditioning (reset conditions)
  ValveAssign : Inport
  FeedPressure : Inport  Port=2
  MainSwitch : Inport  Port=3
  ForceRequest : Inport  Port=4
  BreakLine : ManualSwitch
  BreakLine1 : ManualSwitch
  Bus Creator1 : BusCreator  Inputs=2
  Constant : Constant  Value=0
  Constant1 : Constant
  Data Store Memory : DataStoreMemory  DataStoreName=ShortInGrid  ReadBeforeWriteMsg=warning  WriteAfterWriteMsg=warning  WriteAfterReadMsg=warning  InitialValue=2
  Data Store Read3 : DataStoreRead  DataStoreName=ShortInGrid  SampleTime=0
  Data Store Read6 : DataStoreRead  DataStoreName=ShortInGrid  SampleTime=0
  Data Store Write3 : DataStoreWrite  DataStoreName=ShortInGrid
  Demux : Demux
  FlowIn : Constant
  ForceShort : Subsystem
  IsVenting : MATLABFcn  MATLABFcn=IsVenting  OutputDimensions=1
  IsVenting1 : MATLABFcn  MATLABFcn=IsVenting  OutputDimensions=1
  Manual Switch : ManualSwitch
  Mux : Mux  Inputs=3
  Mux1 : Mux  Inputs=2
  Mux2 : Mux  Inputs=2
  Mux3 : Mux  Inputs=2
  NoFlow : Constant  Value=0
  NoFlow1 : Constant  Value=0
  NoFlow2 : Constant  Value=0
  Off{,2,4,6,8} (5 alike) : Constant  Value=0
  Pressure : MATLABFcn  MATLABFcn=ResultingPressure
  Switch : Switch  Threshold=0.1
  Switch8 : MultiPortSwitch  Inputs=2
  ThrustBlock : Subsystem
  Valve{1..4} (4 alike) : MultiPortSwitch  Inputs=2
  efficiency : Constant
  L1Vent : Outport
  L2Vent : Outport  Port=2
  Forces : Outport  Port=3
  ThrusterData : Outport  Port=4
  wires:
  [MainSwitch] -> Switch8/1, ThrustBlock/3(MainSwitch)
  Valve4/1 -> Mux3/2
  MainSwitch/1 -> [MainSwitch]
  FeedPressure/1 -> Valve3/3, Valve1/3
  IsVenting/1 -> [V2]
  IsVenting1/1 -> [V1]
  Pressure/1 -> Mux/3, Switch/2
  Mux2/1 -> IsVenting/1
  Mux1/1 -> IsVenting1/1
  Bus Creator1/1 -> ThrusterData/1
  ForceRequest/1 -> ThrustBlock/1(ForceRequest)
  [CathodeEfficiency] -> ThrustBlock/5(CathodeEfficiency)
  BreakLine1/1 -> Mux/2, Valve4/3, Mux2/1
  Valve3/1 -> Mux2/2, BreakLine1/1
  NoFlow2/1 -> BreakLine1/2
  Mux/1 -> Bus Creator1/1  "LinePressures"
  Switch/1 -> Switch8/3
  Off8/1 -> Switch8/2
  Off6/1 -> Valve4/2
  Off2/1 -> Valve3/2
  Off4/1 -> Valve2/2
  Off/1 -> Valve1/2
  NoFlow1/1 -> BreakLine/2
  ThrustBlock/1(OutputForce) -> Forces/1
  ThrustBlock/2(ThrusterData) -> Bus Creator1/2  "A1TX1"
  Demux/4 -> Valve4/1
  Demux/3 -> Valve3/1
  Demux/2 -> Valve2/1
  Demux/1 -> Valve1/1
  ValveAssign/1 -> Demux/1
  Data Store Read6/1 -> ThrustBlock/2(Short?)
  Switch8/1 -> ThrustBlock/4(Feed)
  NoFlow/1 -> Switch/3
  FlowIn/1 -> Switch/1
  BreakLine/1 -> Mux/1, Valve2/3, Mux1/1
  Mux3/1 -> Pressure/1
  Valve2/1 -> Mux3/1
  Valve1/1 -> Mux1/2, BreakLine/1
  efficiency/1 -> [CathodeEfficiency]
  [MainSwitch] -> ForceShort/3(MainSwitch)
  Data Store Read3/1 -> ForceShort/2(SC)
  Manual Switch/1 -> ForceShort/1(Event)
  Constant1/1 -> Manual Switch/2
  Constant/1 -> Manual Switch/1
  ForceShort/1(SC_out) -> Data Store Write3/1
  [V1] -> L1Vent/1
  [V2] -> L2Vent/1

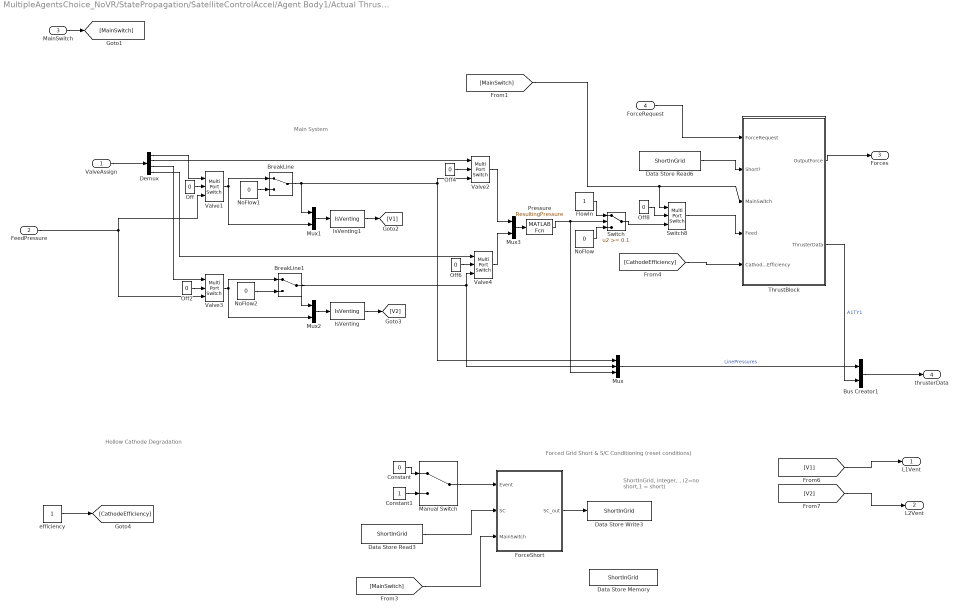
== system MultipleAgentsChoice_NoVR/StatePropagation/SatelliteControlAccel/Agent Body1/Actual Thruster response/Ythruster1/Thruster1 ==
  note: Forced Grid Short & S/C Conditioning (reset conditions)
  note: ShortInGrid, integer, , (2=no short,1 = short)
  note: Hollow Cathode Degradation
  note: Main System
  ValveAssign : Inport
  FeedPressure : Inport  Port=2
  MainSwitch : Inport  Port=3
  ForceRequest : Inport  Port=4
  BreakLine : ManualSwitch
  BreakLine1 : ManualSwitch
  Bus Creator1 : BusCreator  Inputs=2
  Constant : Constant  Value=0
  Constant1 : Constant
  Data Store Memory : DataStoreMemory  DataStoreName=ShortInGrid  ReadBeforeWriteMsg=warning  WriteAfterWriteMsg=warning  WriteAfterReadMsg=warning  InitialValue=2
  Data Store Read3 : DataStoreRead  DataStoreName=ShortInGrid  SampleTime=0
  Data Store Read6 : DataStoreRead  DataStoreName=ShortInGrid  SampleTime=0
  Data Store Write3 : DataStoreWrite  DataStoreName=ShortInGrid
  Demux : Demux
  FlowIn : Constant
  ForceShort : Subsystem
  IsVenting : MATLABFcn  MATLABFcn=IsVenting  OutputDimensions=1
  IsVenting1 : MATLABFcn  MATLABFcn=IsVenting  OutputDimensions=1
  Manual Switch : ManualSwitch
  Mux : Mux  Inputs=3
  Mux1 : Mux  Inputs=2
  Mux2 : Mux  Inputs=2
  Mux3 : Mux  Inputs=2
  NoFlow : Constant  Value=0
  NoFlow1 : Constant  Value=0
  NoFlow2 : Constant  Value=0
  Off{,2,4,6,8} (5 alike) : Constant  Value=0
  Pressure : MATLABFcn  MATLABFcn=ResultingPressure
  Switch : Switch  Threshold=0.1
  Switch8 : MultiPortSwitch  Inputs=2
  ThrustBlock : Subsystem
  Valve{1..4} (4 alike) : MultiPortSwitch  Inputs=2
  efficiency : Constant
  L1Vent : Outport
  L2Vent : Outport  Port=2
  Forces : Outport  Port=3
  thrusterData : Outport  Port=4
  wires:
  ForceShort/1(SC_out) -> Data Store Write3/1
  Constant/1 -> Manual Switch/1
  Constant1/1 -> Manual Switch/2
  Manual Switch/1 -> ForceShort/1(Event)
  Data Store Read3/1 -> ForceShort/2(SC)
  [MainSwitch] -> ForceShort/3(MainSwitch)
  efficiency/1 -> [CathodeEfficiency]
  Valve1/1 -> BreakLine/1, Mux1/2
  Valve2/1 -> Mux3/1
  Mux3/1 -> Pressure/1
  BreakLine/1 -> Mux1/1, Valve2/3, Mux/1
  FlowIn/1 -> Switch/1
  NoFlow/1 -> Switch/3
  Switch8/1 -> ThrustBlock/4(Feed)
  Data Store Read6/1 -> ThrustBlock/2(Short?)
  ValveAssign/1 -> Demux/1
  Demux/1 -> Valve1/1
  Demux/2 -> Valve2/1
  Demux/3 -> Valve3/1
  Demux/4 -> Valve4/1
  ThrustBlock/2(ThrusterData) -> Bus Creator1/2  "A1TY1"
  ThrustBlock/1(OutputForce) -> Forces/1
  NoFlow1/1 -> BreakLine/2
  Off/1 -> Valve1/2
  Off4/1 -> Valve2/2
  Off2/1 -> Valve3/2
  Off6/1 -> Valve4/2
  Off8/1 -> Switch8/2
  Switch/1 -> Switch8/3
  Mux/1 -> Bus Creator1/1  "LinePressures"
  NoFlow2/1 -> BreakLine1/2
  Valve3/1 -> BreakLine1/1, Mux2/2
  BreakLine1/1 -> Mux2/1, Valve4/3, Mux/2
  [CathodeEfficiency] -> ThrustBlock/5(CathodeEfficiency)
  ForceRequest/1 -> ThrustBlock/1(ForceRequest)
  Bus Creator1/1 -> thrusterData/1
  Mux1/1 -> IsVenting1/1
  Mux2/1 -> IsVenting/1
  Pressure/1 -> Switch/2, Mux/3
  IsVenting1/1 -> [V1]
  IsVenting/1 -> [V2]
  FeedPressure/1 -> Valve1/3, Valve3/3
  MainSwitch/1 -> [MainSwitch]
  Valve4/1 -> Mux3/2
  [MainSwitch] -> Switch8/1, ThrustBlock/3(MainSwitch)
  [V1] -> L1Vent/1
  [V2] -> L2Vent/1

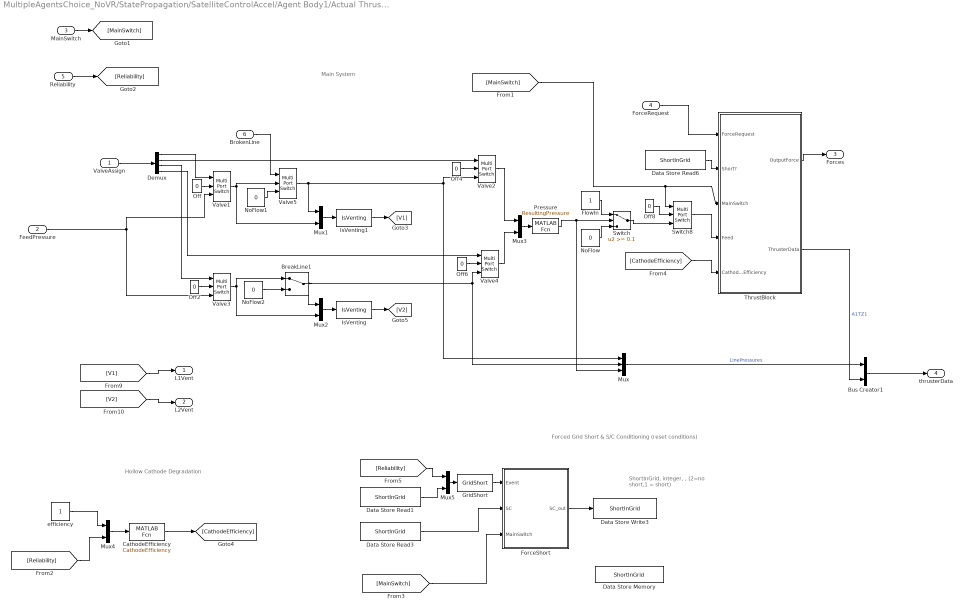
== system MultipleAgentsChoice_NoVR/StatePropagation/SatelliteControlAccel/Agent Body1/Actual Thruster response/Zthruster1/Thruster1 ==
  note: Main System
  note: Hollow Cathode Degradation
  note: ShortInGrid, integer, , (2=no short,1 = short)
  note: Forced Grid Short & S/C Conditioning (reset conditions)
  ValveAssign : Inport
  FeedPressure : Inport  Port=2
  MainSwitch : Inport  Port=3
  ForceRequest : Inport  Port=4
  Reliability : Inport  Port=5
  BrokenLine : Inport  Port=6
  BreakLine1 : ManualSwitch
  Bus Creator1 : BusCreator  Inputs=2
  CathodeEfficiency : MATLABFcn  MATLABFcn=CathodeEfficiency  OutputDimensions=1
  Data Store Memory : DataStoreMemory  DataStoreName=ShortInGrid  ReadBeforeWriteMsg=warning  WriteAfterWriteMsg=warning  WriteAfterReadMsg=warning  InitialValue=2
  Data Store Read1 : DataStoreRead  DataStoreName=ShortInGrid  SampleTime=0
  Data Store Read3 : DataStoreRead  DataStoreName=ShortInGrid  SampleTime=0
  Data Store Read6 : DataStoreRead  DataStoreName=ShortInGrid  SampleTime=0
  Data Store Write3 : DataStoreWrite  DataStoreName=ShortInGrid
  Demux : Demux
  FlowIn : Constant
  ForceShort : Subsystem
  GridShort : MATLABFcn  MATLABFcn=GridShort  OutputDimensions=1
  IsVenting : MATLABFcn  MATLABFcn=IsVenting  OutputDimensions=1
  IsVenting1 : MATLABFcn  MATLABFcn=IsVenting  OutputDimensions=1
  Mux : Mux  Inputs=3
  Mux{1..5} (5 alike) : Mux  Inputs=2
  NoFlow : Constant  Value=0
  NoFlow1 : Constant  Value=0
  NoFlow2 : Constant  Value=0
  Off{,2,4,6,8} (5 alike) : Constant  Value=0
  Pressure : MATLABFcn  MATLABFcn=ResultingPressure
  Switch : Switch  Threshold=0.1
  Switch8 : MultiPortSwitch  Inputs=2
  ThrustBlock : Subsystem
  Valve{1..5} (5 alike) : MultiPortSwitch  Inputs=2
  efficiency : Constant
  L1Vent : Outport
  L2Vent : Outport  Port=2
  Forces : Outport  Port=3
  thrusterData : Outport  Port=4
  wires:
  BrokenLine/1 -> Valve5/1
  [Reliability] -> Mux5/1
  Data Store Read1/1 -> Mux5/2
  Mux5/1 -> GridShort/1
  CathodeEfficiency/1 -> [CathodeEfficiency]
  Mux4/1 -> CathodeEfficiency/1
  [Reliability] -> Mux4/2
  efficiency/1 -> Mux4/1
  Reliability/1 -> [Reliability]
  [MainSwitch] -> Switch8/1, ThrustBlock/3(MainSwitch)
  Valve4/1 -> Mux3/2
  MainSwitch/1 -> [MainSwitch]
  FeedPressure/1 -> Valve3/3, Valve1/3
  IsVenting/1 -> [V2]
  IsVenting1/1 -> [V1]
  Pressure/1 -> Mux/3, Switch/2
  Mux2/1 -> IsVenting/1
  Mux1/1 -> IsVenting1/1
  Bus Creator1/1 -> thrusterData/1
  ForceRequest/1 -> ThrustBlock/1(ForceRequest)
  [CathodeEfficiency] -> ThrustBlock/5(CathodeEfficiency)
  BreakLine1/1 -> Mux/2, Valve4/3, Mux2/1
  Valve3/1 -> Mux2/2, BreakLine1/1
  NoFlow2/1 -> BreakLine1/2
  Mux/1 -> Bus Creator1/1  "LinePressures"
  Switch/1 -> Switch8/3
  Off8/1 -> Switch8/2
  Off6/1 -> Valve4/2
  Off2/1 -> Valve3/2
  Off4/1 -> Valve2/2
  Off/1 -> Valve1/2
  NoFlow1/1 -> Valve5/3
  ThrustBlock/1(OutputForce) -> Forces/1
  ThrustBlock/2(ThrusterData) -> Bus Creator1/2  "A1TZ1"
  Demux/4 -> Valve4/1
  Demux/3 -> Valve3/1
  Demux/2 -> Valve2/1
  Demux/1 -> Valve1/1
  ValveAssign/1 -> Demux/1
  Data Store Read6/1 -> ThrustBlock/2(Short?)
  Switch8/1 -> ThrustBlock/4(Feed)
  NoFlow/1 -> Switch/3
  FlowIn/1 -> Switch/1
  Valve5/1 -> Mux/1, Valve2/3, Mux1/1
  Mux3/1 -> Pressure/1
  Valve2/1 -> Mux3/1
  Valve1/1 -> Mux1/2, Valve5/2
  [MainSwitch] -> ForceShort/3(MainSwitch)
  Data Store Read3/1 -> ForceShort/2(SC)
  GridShort/1 -> ForceShort/1(Event)
  ForceShort/1(SC_out) -> Data Store Write3/1
  [V1] -> L1Vent/1
  [V2] -> L2Vent/1
